simulink model "testsiggen"  (R2018a)
settings: Solver=VariableStepAuto  StartTime=0.0  StopTime=10.0  RelTol=1e-3
model workspace (MAT data in the model file):
  J = 0.14
  p = [-0.0001 0.1 0 0 0.1]
  spe_speed_sdosession = sldodialogs.data.SessionData
  spe_speed_sdosession.Version = '3.0'
  spe_speed_sdosession.Data.ModelName = 'spe_speed'
  spe_speed_sdosession.Data.ToolType = 'ParameterEstimation'
  spe_speed_sdosession.Data.GUIOptions.NoPromptClose = 0
  spe_speed_sdosession.Data.Workspace.LocalWorkspace.EstimationData = sdo.Experiment
  spe_speed_sdosession.Data.Workspace.LocalWorkspace.EstimationData.ModelName = 'spe_speed'
  spe_speed_sdosession.Data.Workspace.LocalWorkspace.EstimationData.InputData = Simulink.SimulationData.Signal
  spe_speed_sdosession.Data.Workspace.LocalWorkspace.EstimationData.InputData.BlockPath = Simulink.SimulationData.BlockPath
  spe_speed_sdosession.Data.Workspace.LocalWorkspace.EstimationData.InputData.BlockPath.path = {'spe_speed/Throttle'}
  spe_speed_sdosession.Data.Workspace.LocalWorkspace.EstimationData.InputData.Values = timeseries
  spe_speed_sdosession.Data.Workspace.LocalWorkspace.EstimationData.InputData.Values.Name = 'spe_speed/Throttle:1'
  spe_speed_sdosession.Data.Workspace.LocalWorkspace.EstimationData.InputData.Values.DataInfo = tsdata.datametadata
  spe_speed_sdosession.Data.Workspace.LocalWorkspace.EstimationData.InputData.Values.DataInfo.Interpolation = tsdata.interpolation
  spe_speed_sdosession.Data.Workspace.LocalWorkspace.EstimationData.InputData.Values.DataInfo.Interpolation.Fhandle : function handle (value not decoded)
  spe_speed_sdosession.Data.Workspace.LocalWorkspace.EstimationData.InputData.Values.DataInfo.Interpolation.Name = 'linear'
  spe_speed_sdosession.Data.Workspace.LocalWorkspace.EstimationData.InputData.Values.TimeInfo = tsdata.timemetadata
  spe_speed_sdosession.Data.Workspace.LocalWorkspace.EstimationData.InputData.Values.TimeInfo.Length = 804
  spe_speed_sdosession.Data.Workspace.LocalWorkspace.EstimationData.InputData.Values.TimeInfo.DuplicateTimes = 0
  spe_speed_sdosession.Data.Workspace.LocalWorkspace.EstimationData.InputData.Values.TimeInfo.Time_ = [0 0.05 0.1 0.15 0.2 0.25 0.3 0.35 0.4 0.45 0.5 0.55 ... (804 elements, 804x1)]
  spe_speed_sdosession.Data.Workspace.LocalWorkspace.EstimationData.InputData.Values.TimeInfo.Initialized = 1
  spe_speed_sdosession.Data.Workspace.LocalWorkspace.EstimationData.InputData.Values.QualityInfo = tsdata.qualmetadata
  spe_speed_sdosession.Data.Workspace.LocalWorkspace.EstimationData.InputData.Values.Data_ = [8.973 8.973 8.973 8.973 8.973 8.973 8.973 8.973 8.973 8.973 8.973 8.973 ... (804 elements, 804x1)]
  spe_speed_sdosession.Data.Workspace.LocalWorkspace.EstimationData.InputData.Name = 'spe_speed/Throttle:1'
  spe_speed_sdosession.Data.Workspace.LocalWorkspace.EstimationData.OutputData = Simulink.SimulationData.Signal
  spe_speed_sdosession.Data.Workspace.LocalWorkspace.EstimationData.OutputData.PortType = 'outport'
  spe_speed_sdosession.Data.Workspace.LocalWorkspace.EstimationData.OutputData.BlockPath = Simulink.SimulationData.BlockPath
  spe_speed_sdosession.Data.Workspace.LocalWorkspace.EstimationData.OutputData.BlockPath.path = {'spe_speed/rad//s to rpm'}
  spe_speed_sdosession.Data.Workspace.LocalWorkspace.EstimationData.OutputData.Values = timeseries
  spe_speed_sdosession.Data.Workspace.LocalWorkspace.EstimationData.OutputData.Values.Name = 'spe_speed/rad//s to rpm:1'
  spe_speed_sdosession.Data.Workspace.LocalWorkspace.EstimationData.OutputData.Values.DataInfo = tsdata.datametadata
  spe_speed_sdosession.Data.Workspace.LocalWorkspace.EstimationData.OutputData.Values.DataInfo.Interpolation = tsdata.interpolation
  spe_speed_sdosession.Data.Workspace.LocalWorkspace.EstimationData.OutputData.Values.DataInfo.Interpolation.Fhandle : function handle (value not decoded)
  spe_speed_sdosession.Data.Workspace.LocalWorkspace.EstimationData.OutputData.Values.DataInfo.Interpolation.Name = 'linear'
  spe_speed_sdosession.Data.Workspace.LocalWorkspace.EstimationData.OutputData.Values.TimeInfo = tsdata.timemetadata
  spe_speed_sdosession.Data.Workspace.LocalWorkspace.EstimationData.OutputData.Values.TimeInfo.Length = 804
  spe_speed_sdosession.Data.Workspace.LocalWorkspace.EstimationData.OutputData.Values.TimeInfo.DuplicateTimes = 0
  spe_speed_sdosession.Data.Workspace.LocalWorkspace.EstimationData.OutputData.Values.TimeInfo.Time_ = [0 0.05 0.1 0.15 0.2 0.25 0.3 0.35 0.4 0.45 0.5 0.55 ... (804 elements, 804x1)]
  spe_speed_sdosession.Data.Workspace.LocalWorkspace.EstimationData.OutputData.Values.TimeInfo.Initialized = 1
  spe_speed_sdosession.Data.Workspace.LocalWorkspace.EstimationData.OutputData.Values.QualityInfo = tsdata.qualmetadata
  spe_speed_sdosession.Data.Workspace.LocalWorkspace.EstimationData.OutputData.Values.Data_ = [2005.2 2032.3 1988.5 2017.4 2002.7 1994.8 1987.6 2001.9 2007.9 2003.5 2007.1 2006.9 ... (804 elements, 804x1)]
  spe_speed_sdosession.Data.Workspace.LocalWorkspace.EstimationData.OutputData.Name = 'spe_speed/rad//s to rpm:1'
  spe_speed_sdosession.Data.Workspace.LocalWorkspace.EstimationData.Name = 'EstimationData'
  spe_speed_sdosession.Data.Workspace.LocalWorkspace.ValidationData = sdo.Experiment
  spe_speed_sdosession.Data.Workspace.LocalWorkspace.ValidationData.ModelName = 'spe_speed'
  spe_speed_sdosession.Data.Workspace.LocalWorkspace.ValidationData.InputData = Simulink.SimulationData.Signal
  spe_speed_sdosession.Data.Workspace.LocalWorkspace.ValidationData.InputData.BlockPath = Simulink.SimulationData.BlockPath
  spe_speed_sdosession.Data.Workspace.LocalWorkspace.ValidationData.InputData.BlockPath.path = {'spe_speed/Throttle'}
  spe_speed_sdosession.Data.Workspace.LocalWorkspace.ValidationData.InputData.Values = timeseries
  spe_speed_sdosession.Data.Workspace.LocalWorkspace.ValidationData.InputData.Values.Name = 'unnamed'
  spe_speed_sdosession.Data.Workspace.LocalWorkspace.ValidationData.InputData.Values.DataInfo = tsdata.datametadata
  spe_speed_sdosession.Data.Workspace.LocalWorkspace.ValidationData.InputData.Values.DataInfo.Interpolation = tsdata.interpolation
  spe_speed_sdosession.Data.Workspace.LocalWorkspace.ValidationData.InputData.Values.DataInfo.Interpolation.Fhandle : function handle (value not decoded)
  spe_speed_sdosession.Data.Workspace.LocalWorkspace.ValidationData.InputData.Values.DataInfo.Interpolation.Name = 'linear'
  spe_speed_sdosession.Data.Workspace.LocalWorkspace.ValidationData.InputData.Values.TimeInfo = tsdata.timemetadata
  spe_speed_sdosession.Data.Workspace.LocalWorkspace.ValidationData.InputData.Values.TimeInfo.Length = 801
  spe_speed_sdosession.Data.Workspace.LocalWorkspace.ValidationData.InputData.Values.TimeInfo.DuplicateTimes = 0
  spe_speed_sdosession.Data.Workspace.LocalWorkspace.ValidationData.InputData.Values.TimeInfo.Time_ = [0 0.05 0.1 0.15 0.2 0.25 0.3 0.35 0.4 0.45 0.5 0.55 ... (801 elements, 801x1)]
  spe_speed_sdosession.Data.Workspace.LocalWorkspace.ValidationData.InputData.Values.TimeInfo.Initialized = 1
  spe_speed_sdosession.Data.Workspace.LocalWorkspace.ValidationData.InputData.Values.QualityInfo = tsdata.qualmetadata
  spe_speed_sdosession.Data.Workspace.LocalWorkspace.ValidationData.InputData.Values.Data_ = [8.973 8.9734 8.974 8.9748 8.9758 8.977 8.9784 8.98 8.9818 8.9838 8.9859 8.9883 ... (801 elements, 801x1)]
  spe_speed_sdosession.Data.Workspace.LocalWorkspace.ValidationData.OutputData = Simulink.SimulationData.Signal
  spe_speed_sdosession.Data.Workspace.LocalWorkspace.ValidationData.OutputData.PortType = 'outport'
  spe_speed_sdosession.Data.Workspace.LocalWorkspace.ValidationData.OutputData.BlockPath = Simulink.SimulationData.BlockPath
  spe_speed_sdosession.Data.Workspace.LocalWorkspace.ValidationData.OutputData.BlockPath.path = {'spe_speed/rad//s to rpm'}
  spe_speed_sdosession.Data.Workspace.LocalWorkspace.ValidationData.OutputData.Values = timeseries
  spe_speed_sdosession.Data.Workspace.LocalWorkspace.ValidationData.OutputData.Values.Name = 'unnamed'
  spe_speed_sdosession.Data.Workspace.LocalWorkspace.ValidationData.OutputData.Values.DataInfo = tsdata.datametadata
  spe_speed_sdosession.Data.Workspace.LocalWorkspace.ValidationData.OutputData.Values.DataInfo.Interpolation = tsdata.interpolation
  spe_speed_sdosession.Data.Workspace.LocalWorkspace.ValidationData.OutputData.Values.DataInfo.Interpolation.Fhandle : function handle (value not decoded)
  spe_speed_sdosession.Data.Workspace.LocalWorkspace.ValidationData.OutputData.Values.DataInfo.Interpolation.Name = 'linear'
  spe_speed_sdosession.Data.Workspace.LocalWorkspace.ValidationData.OutputData.Values.TimeInfo = tsdata.timemetadata
  spe_speed_sdosession.Data.Workspace.LocalWorkspace.ValidationData.OutputData.Values.TimeInfo.Length = 801
  spe_speed_sdosession.Data.Workspace.LocalWorkspace.ValidationData.OutputData.Values.TimeInfo.DuplicateTimes = 0
  spe_speed_sdosession.Data.Workspace.LocalWorkspace.ValidationData.OutputData.Values.TimeInfo.Time_ = [0 0.05 0.1 0.15 0.2 0.25 0.3 0.35 0.4 0.45 0.5 0.55 ... (801 elements, 801x1)]
  spe_speed_sdosession.Data.Workspace.LocalWorkspace.ValidationData.OutputData.Values.TimeInfo.Initialized = 1
  spe_speed_sdosession.Data.Workspace.LocalWorkspace.ValidationData.OutputData.Values.QualityInfo = tsdata.qualmetadata
  spe_speed_sdosession.Data.Workspace.LocalWorkspace.ValidationData.OutputData.Values.Data_ = [2005.2 2032.3 1988.5 2017.4 2002.7 1994.9 1987.8 2002.1 2008.2 2004 2007.7 2007.7 ... (801 elements, 801x1)]
  spe_speed_sdosession.Data.Workspace.LocalWorkspace.ValidationData.Name = 'ValidationData'
  spe_speed_sdosession.Data.Workspace.HiddenWorkspace.EstimatedParams = param.Continuous
  spe_speed_sdosession.Data.Workspace.HiddenWorkspace.EstimatedParams.Scale_ = [-0.0001 0.1 0 0 0.1]
  spe_speed_sdosession.Data.Workspace.HiddenWorkspace.EstimatedParams.Size_ = [1 5]
  spe_speed_sdosession.Data.Workspace.HiddenWorkspace.EstimatedParams.Value_ = [-0.0001 0.1 0 0 0.1]
  spe_speed_sdosession.Data.Workspace.HiddenWorkspace.EstimatedParams.pID = paramid.Variable
  spe_speed_sdosession.Data.Workspace.HiddenWorkspace.EstimatedParams.pID.Name = 'p'
  spe_speed_sdosession.Data.Workspace.HiddenWorkspace.UVars = []
  spe_speed_sdosession.Data.ToolData.PlotManager.Plots.Class = 'sldoplots.ExperimentPlot'
  spe_speed_sdosession.Data.ToolData.PlotManager.Plots.Sources = {'EstimationData'}
  spe_speed_sdosession.Data.ToolData.DialogManager = []
  spe_speed_sdosession.Data.ToolData.ParameterEstimation.DesignVariables = 'EstimatedParams'
  spe_speed_sdosession.Data.ToolData.ParameterEstimation.UncertainVariables = 'UVars'
  spe_speed_sdosession.Data.ToolData.ParameterEstimation.Options = sdo.OptimizeOptions
  spe_speed_sdosession.Data.ToolData.ParameterEstimation.Options.Method = 'lsqnonlin'
  spe_speed_sdosession.Data.ToolData.ParameterEstimation.Options.MethodOptions = optim.options.Lsqnonlin
  spe_speed_sdosession.Data.ToolData.ParameterEstimation.Options.MethodOptions.LsqnonlinVersion = 4
  spe_speed_sdosession.Data.ToolData.ParameterEstimation.Options.MethodOptions.OptionsStore.AlgorithmNames = {'trust-region-reflective', 'levenberg-marquardt'}
  spe_speed_sdosession.Data.ToolData.ParameterEstimation.Options.MethodOptions.OptionsStore.DefaultAlgorithm = 'trust-region-reflective'
  spe_speed_sdosession.Data.ToolData.ParameterEstimation.Options.MethodOptions.OptionsStore.AlgorithmDefaults{1}.DerivativeCheck = 'off'
  spe_speed_sdosession.Data.ToolData.ParameterEstimation.Options.MethodOptions.OptionsStore.AlgorithmDefaults{1}.Diagnostics = 'off'
  spe_speed_sdosession.Data.ToolData.ParameterEstimation.Options.MethodOptions.OptionsStore.AlgorithmDefaults{1}.DiffMaxChange = Inf
  spe_speed_sdosession.Data.ToolData.ParameterEstimation.Options.MethodOptions.OptionsStore.AlgorithmDefaults{1}.DiffMinChange = 0
  spe_speed_sdosession.Data.ToolData.ParameterEstimation.Options.MethodOptions.OptionsStore.AlgorithmDefaults{1}.Display = 'final'
  spe_speed_sdosession.Data.ToolData.ParameterEstimation.Options.MethodOptions.OptionsStore.AlgorithmDefaults{1}.FinDiffRelStep = 'sqrt(eps)'
  spe_speed_sdosession.Data.ToolData.ParameterEstimation.Options.MethodOptions.OptionsStore.AlgorithmDefaults{1}.FinDiffType = 'forward'
  spe_speed_sdosession.Data.ToolData.ParameterEstimation.Options.MethodOptions.OptionsStore.AlgorithmDefaults{1}.FunValCheck = 'off'
  spe_speed_sdosession.Data.ToolData.ParameterEstimation.Options.MethodOptions.OptionsStore.AlgorithmDefaults{1}.Jacobian = 'off'
  spe_speed_sdosession.Data.ToolData.ParameterEstimation.Options.MethodOptions.OptionsStore.AlgorithmDefaults{1}.MaxFunEvals = '100*numberOfVariables'
  spe_speed_sdosession.Data.ToolData.ParameterEstimation.Options.MethodOptions.OptionsStore.AlgorithmDefaults{1}.MaxIter = 400
  spe_speed_sdosession.Data.ToolData.ParameterEstimation.Options.MethodOptions.OptionsStore.AlgorithmDefaults{1}.OutputFcn = []
  spe_speed_sdosession.Data.ToolData.ParameterEstimation.Options.MethodOptions.OptionsStore.AlgorithmDefaults{1}.PlotFcns = []
  spe_speed_sdosession.Data.ToolData.ParameterEstimation.Options.MethodOptions.OptionsStore.AlgorithmDefaults{1}.TolFunValue = 1e-06
  spe_speed_sdosession.Data.ToolData.ParameterEstimation.Options.MethodOptions.OptionsStore.AlgorithmDefaults{1}.TolFun = 1e-06
  spe_speed_sdosession.Data.ToolData.ParameterEstimation.Options.MethodOptions.OptionsStore.AlgorithmDefaults{1}.TolX = 1e-06
  spe_speed_sdosession.Data.ToolData.ParameterEstimation.Options.MethodOptions.OptionsStore.AlgorithmDefaults{1}.TypicalX = 'ones(numberOfVariables,1)'
  spe_speed_sdosession.Data.ToolData.ParameterEstimation.Options.MethodOptions.OptionsStore.AlgorithmDefaults{1}.JacobMult = []
  spe_speed_sdosession.Data.ToolData.ParameterEstimation.Options.MethodOptions.OptionsStore.AlgorithmDefaults{1}.JacobPattern = 'sparse(ones(Jrows,Jcols))'
  spe_speed_sdosession.Data.ToolData.ParameterEstimation.Options.MethodOptions.OptionsStore.AlgorithmDefaults{1}.MaxPCGIter = 'max(1,floor(numberOfVariables/2))'
  spe_speed_sdosession.Data.ToolData.ParameterEstimation.Options.MethodOptions.OptionsStore.AlgorithmDefaults{1}.PrecondBandWidth = Inf
  spe_speed_sdosession.Data.ToolData.ParameterEstimation.Options.MethodOptions.OptionsStore.AlgorithmDefaults{1}.TolPCG = 0.1
  spe_speed_sdosession.Data.ToolData.ParameterEstimation.Options.MethodOptions.OptionsStore.AlgorithmDefaults{1}.UseParallel = 0
  spe_speed_sdosession.Data.ToolData.ParameterEstimation.Options.MethodOptions.OptionsStore.AlgorithmDefaults{2}.DerivativeCheck = 'off'
  spe_speed_sdosession.Data.ToolData.ParameterEstimation.Options.MethodOptions.OptionsStore.AlgorithmDefaults{2}.Diagnostics = 'off'
  spe_speed_sdosession.Data.ToolData.ParameterEstimation.Options.MethodOptions.OptionsStore.AlgorithmDefaults{2}.DiffMaxChange = Inf
  spe_speed_sdosession.Data.ToolData.ParameterEstimation.Options.MethodOptions.OptionsStore.AlgorithmDefaults{2}.DiffMinChange = 0
  spe_speed_sdosession.Data.ToolData.ParameterEstimation.Options.MethodOptions.OptionsStore.AlgorithmDefaults{2}.Display = 'final'
  spe_speed_sdosession.Data.ToolData.ParameterEstimation.Options.MethodOptions.OptionsStore.AlgorithmDefaults{2}.FinDiffRelStep = 'sqrt(eps)'
  spe_speed_sdosession.Data.ToolData.ParameterEstimation.Options.MethodOptions.OptionsStore.AlgorithmDefaults{2}.FinDiffType = 'forward'
  spe_speed_sdosession.Data.ToolData.ParameterEstimation.Options.MethodOptions.OptionsStore.AlgorithmDefaults{2}.FunValCheck = 'off'
  spe_speed_sdosession.Data.ToolData.ParameterEstimation.Options.MethodOptions.OptionsStore.AlgorithmDefaults{2}.Jacobian = 'off'
  spe_speed_sdosession.Data.ToolData.ParameterEstimation.Options.MethodOptions.OptionsStore.AlgorithmDefaults{2}.InitDamping = 0.01
  spe_speed_sdosession.Data.ToolData.ParameterEstimation.Options.MethodOptions.OptionsStore.AlgorithmDefaults{2}.MaxFunEvals = '200*numberOfVariables'
  spe_speed_sdosession.Data.ToolData.ParameterEstimation.Options.MethodOptions.OptionsStore.AlgorithmDefaults{2}.MaxIter = 400
  spe_speed_sdosession.Data.ToolData.ParameterEstimation.Options.MethodOptions.OptionsStore.AlgorithmDefaults{2}.OutputFcn = []
  spe_speed_sdosession.Data.ToolData.ParameterEstimation.Options.MethodOptions.OptionsStore.AlgorithmDefaults{2}.PlotFcns = []
  spe_speed_sdosession.Data.ToolData.ParameterEstimation.Options.MethodOptions.OptionsStore.AlgorithmDefaults{2}.TolFunValue = 1e-06
  spe_speed_sdosession.Data.ToolData.ParameterEstimation.Options.MethodOptions.OptionsStore.AlgorithmDefaults{2}.TolX = 1e-06
  spe_speed_sdosession.Data.ToolData.ParameterEstimation.Options.MethodOptions.OptionsStore.AlgorithmDefaults{2}.TypicalX = 'ones(numberOfVariables,1)'
  spe_speed_sdosession.Data.ToolData.ParameterEstimation.Options.MethodOptions.OptionsStore.AlgorithmDefaults{2}.ScaleProblem = 'none'
  spe_speed_sdosession.Data.ToolData.ParameterEstimation.Options.MethodOptions.OptionsStore.AlgorithmDefaults{2}.UseParallel = 0
  spe_speed_sdosession.Data.ToolData.ParameterEstimation.Options.MethodOptions.OptionsStore.AlgorithmIndex = [1 0]
  spe_speed_sdosession.Data.ToolData.ParameterEstimation.Options.MethodOptions.OptionsStore.SetByUser.DerivativeCheck = 0
  spe_speed_sdosession.Data.ToolData.ParameterEstimation.Options.MethodOptions.OptionsStore.SetByUser.Diagnostics = 0
  spe_speed_sdosession.Data.ToolData.ParameterEstimation.Options.MethodOptions.OptionsStore.SetByUser.DiffMaxChange = 0
  spe_speed_sdosession.Data.ToolData.ParameterEstimation.Options.MethodOptions.OptionsStore.SetByUser.DiffMinChange = 0
  spe_speed_sdosession.Data.ToolData.ParameterEstimation.Options.MethodOptions.OptionsStore.SetByUser.Display = 1
  spe_speed_sdosession.Data.ToolData.ParameterEstimation.Options.MethodOptions.OptionsStore.SetByUser.FinDiffRelStep = 0
  spe_speed_sdosession.Data.ToolData.ParameterEstimation.Options.MethodOptions.OptionsStore.SetByUser.FinDiffType = 0
  spe_speed_sdosession.Data.ToolData.ParameterEstimation.Options.MethodOptions.OptionsStore.SetByUser.FunValCheck = 0
  spe_speed_sdosession.Data.ToolData.ParameterEstimation.Options.MethodOptions.OptionsStore.SetByUser.InitDamping = 0
  spe_speed_sdosession.Data.ToolData.ParameterEstimation.Options.MethodOptions.OptionsStore.SetByUser.JacobMult = 0
  spe_speed_sdosession.Data.ToolData.ParameterEstimation.Options.MethodOptions.OptionsStore.SetByUser.JacobPattern = 0
  spe_speed_sdosession.Data.ToolData.ParameterEstimation.Options.MethodOptions.OptionsStore.SetByUser.Jacobian = 1
  spe_speed_sdosession.Data.ToolData.ParameterEstimation.Options.MethodOptions.OptionsStore.SetByUser.MaxFunEvals = 1
  spe_speed_sdosession.Data.ToolData.ParameterEstimation.Options.MethodOptions.OptionsStore.SetByUser.MaxIter = 1
  spe_speed_sdosession.Data.ToolData.ParameterEstimation.Options.MethodOptions.OptionsStore.SetByUser.MaxPCGIter = 0
  spe_speed_sdosession.Data.ToolData.ParameterEstimation.Options.MethodOptions.OptionsStore.SetByUser.OutputFcn = 0
  spe_speed_sdosession.Data.ToolData.ParameterEstimation.Options.MethodOptions.OptionsStore.SetByUser.PlotFcns = 0
  spe_speed_sdosession.Data.ToolData.ParameterEstimation.Options.MethodOptions.OptionsStore.SetByUser.PrecondBandWidth = 0
  spe_speed_sdosession.Data.ToolData.ParameterEstimation.Options.MethodOptions.OptionsStore.SetByUser.ScaleProblem = 0
  spe_speed_sdosession.Data.ToolData.ParameterEstimation.Options.MethodOptions.OptionsStore.SetByUser.TolFun = 1
  spe_speed_sdosession.Data.ToolData.ParameterEstimation.Options.MethodOptions.OptionsStore.SetByUser.TolFunValue = 1
  spe_speed_sdosession.Data.ToolData.ParameterEstimation.Options.MethodOptions.OptionsStore.SetByUser.TolPCG = 0
  spe_speed_sdosession.Data.ToolData.ParameterEstimation.Options.MethodOptions.OptionsStore.SetByUser.TolX = 1
  spe_speed_sdosession.Data.ToolData.ParameterEstimation.Options.MethodOptions.OptionsStore.SetByUser.TypicalX = 0
  spe_speed_sdosession.Data.ToolData.ParameterEstimation.Options.MethodOptions.OptionsStore.SetByUser.UseParallel = 0
  spe_speed_sdosession.Data.ToolData.ParameterEstimation.Options.MethodOptions.OptionsStore.SetByUser.Algorithm = 0
  spe_speed_sdosession.Data.ToolData.ParameterEstimation.Options.MethodOptions.OptionsStore.NonConstantDefaultFields = {'MaxFunEvals'}
  spe_speed_sdosession.Data.ToolData.ParameterEstimation.Options.MethodOptions.OptionsStore.IsConstantDefault.DerivativeCheck = 1
  spe_speed_sdosession.Data.ToolData.ParameterEstimation.Options.MethodOptions.OptionsStore.IsConstantDefault.Diagnostics = 1
  spe_speed_sdosession.Data.ToolData.ParameterEstimation.Options.MethodOptions.OptionsStore.IsConstantDefault.DiffMaxChange = 1
  spe_speed_sdosession.Data.ToolData.ParameterEstimation.Options.MethodOptions.OptionsStore.IsConstantDefault.DiffMinChange = 1
  spe_speed_sdosession.Data.ToolData.ParameterEstimation.Options.MethodOptions.OptionsStore.IsConstantDefault.Display = 1
  spe_speed_sdosession.Data.ToolData.ParameterEstimation.Options.MethodOptions.OptionsStore.IsConstantDefault.FinDiffRelStep = 1
  spe_speed_sdosession.Data.ToolData.ParameterEstimation.Options.MethodOptions.OptionsStore.IsConstantDefault.FinDiffType = 1
  spe_speed_sdosession.Data.ToolData.ParameterEstimation.Options.MethodOptions.OptionsStore.IsConstantDefault.FunValCheck = 1
  spe_speed_sdosession.Data.ToolData.ParameterEstimation.Options.MethodOptions.OptionsStore.IsConstantDefault.InitDamping = 1
  spe_speed_sdosession.Data.ToolData.ParameterEstimation.Options.MethodOptions.OptionsStore.IsConstantDefault.JacobMult = 1
  spe_speed_sdosession.Data.ToolData.ParameterEstimation.Options.MethodOptions.OptionsStore.IsConstantDefault.JacobPattern = 1
  spe_speed_sdosession.Data.ToolData.ParameterEstimation.Options.MethodOptions.OptionsStore.IsConstantDefault.Jacobian = 1
  spe_speed_sdosession.Data.ToolData.ParameterEstimation.Options.MethodOptions.OptionsStore.IsConstantDefault.MaxFunEvals = 0
  spe_speed_sdosession.Data.ToolData.ParameterEstimation.Options.MethodOptions.OptionsStore.IsConstantDefault.MaxIter = 1
  spe_speed_sdosession.Data.ToolData.ParameterEstimation.Options.MethodOptions.OptionsStore.IsConstantDefault.MaxPCGIter = 1
  spe_speed_sdosession.Data.ToolData.ParameterEstimation.Options.MethodOptions.OptionsStore.IsConstantDefault.OutputFcn = 1
  spe_speed_sdosession.Data.ToolData.ParameterEstimation.Options.MethodOptions.OptionsStore.IsConstantDefault.PlotFcns = 1
  spe_speed_sdosession.Data.ToolData.ParameterEstimation.Options.MethodOptions.OptionsStore.IsConstantDefault.PrecondBandWidth = 1
  spe_speed_sdosession.Data.ToolData.ParameterEstimation.Options.MethodOptions.OptionsStore.IsConstantDefault.ScaleProblem = 1
  spe_speed_sdosession.Data.ToolData.ParameterEstimation.Options.MethodOptions.OptionsStore.IsConstantDefault.TolFun = 1
  spe_speed_sdosession.Data.ToolData.ParameterEstimation.Options.MethodOptions.OptionsStore.IsConstantDefault.TolFunValue = 1
  spe_speed_sdosession.Data.ToolData.ParameterEstimation.Options.MethodOptions.OptionsStore.IsConstantDefault.TolPCG = 1
  spe_speed_sdosession.Data.ToolData.ParameterEstimation.Options.MethodOptions.OptionsStore.IsConstantDefault.TolX = 1
  spe_speed_sdosession.Data.ToolData.ParameterEstimation.Options.MethodOptions.OptionsStore.IsConstantDefault.TypicalX = 1
  spe_speed_sdosession.Data.ToolData.ParameterEstimation.Options.MethodOptions.OptionsStore.IsConstantDefault.UseParallel = 1
  spe_speed_sdosession.Data.ToolData.ParameterEstimation.Options.MethodOptions.OptionsStore.IsConstantDefault.Algorithm = 1
  spe_speed_sdosession.Data.ToolData.ParameterEstimation.Options.MethodOptions.OptionsStore.NonConstantDefaults.MaxFunEvals = {'100*numberOfVariables', '200*numberOfVariables'}
  spe_speed_sdosession.Data.ToolData.ParameterEstimation.Options.MethodOptions.OptionsStore.Options.DerivativeCheck = 'off'
  spe_speed_sdosession.Data.ToolData.ParameterEstimation.Options.MethodOptions.OptionsStore.Options.Diagnostics = 'off'
  spe_speed_sdosession.Data.ToolData.ParameterEstimation.Options.MethodOptions.OptionsStore.Options.DiffMaxChange = Inf
  spe_speed_sdosession.Data.ToolData.ParameterEstimation.Options.MethodOptions.OptionsStore.Options.DiffMinChange = 0
  spe_speed_sdosession.Data.ToolData.ParameterEstimation.Options.MethodOptions.OptionsStore.Options.Display = 'iter'
  spe_speed_sdosession.Data.ToolData.ParameterEstimation.Options.MethodOptions.OptionsStore.Options.FinDiffRelStep = 'sqrt(eps)'
  spe_speed_sdosession.Data.ToolData.ParameterEstimation.Options.MethodOptions.OptionsStore.Options.FinDiffType = 'forward'
  spe_speed_sdosession.Data.ToolData.ParameterEstimation.Options.MethodOptions.OptionsStore.Options.FunValCheck = 'off'
  spe_speed_sdosession.Data.ToolData.ParameterEstimation.Options.MethodOptions.OptionsStore.Options.Jacobian = 'on'
  spe_speed_sdosession.Data.ToolData.ParameterEstimation.Options.MethodOptions.OptionsStore.Options.MaxFunEvals = Inf
  spe_speed_sdosession.Data.ToolData.ParameterEstimation.Options.MethodOptions.OptionsStore.Options.MaxIter = 100
  spe_speed_sdosession.Data.ToolData.ParameterEstimation.Options.MethodOptions.OptionsStore.Options.OutputFcn = []
  spe_speed_sdosession.Data.ToolData.ParameterEstimation.Options.MethodOptions.OptionsStore.Options.PlotFcns = []
  spe_speed_sdosession.Data.ToolData.ParameterEstimation.Options.MethodOptions.OptionsStore.Options.TolFunValue = 1e-06
  spe_speed_sdosession.Data.ToolData.ParameterEstimation.Options.MethodOptions.OptionsStore.Options.TolFun = 1e-06
  spe_speed_sdosession.Data.ToolData.ParameterEstimation.Options.MethodOptions.OptionsStore.Options.TolX = 1e-06
  spe_speed_sdosession.Data.ToolData.ParameterEstimation.Options.MethodOptions.OptionsStore.Options.TypicalX = 'ones(numberOfVariables,1)'
  spe_speed_sdosession.Data.ToolData.ParameterEstimation.Options.MethodOptions.OptionsStore.Options.JacobMult = []
  spe_speed_sdosession.Data.ToolData.ParameterEstimation.Options.MethodOptions.OptionsStore.Options.JacobPattern = 'sparse(ones(Jrows,Jcols))'
  spe_speed_sdosession.Data.ToolData.ParameterEstimation.Options.MethodOptions.OptionsStore.Options.MaxPCGIter = 'max(1,floor(numberOfVariables/2))'
  spe_speed_sdosession.Data.ToolData.ParameterEstimation.Options.MethodOptions.OptionsStore.Options.PrecondBandWidth = Inf
  spe_speed_sdosession.Data.ToolData.ParameterEstimation.Options.MethodOptions.OptionsStore.Options.TolPCG = 0.1
  spe_speed_sdosession.Data.ToolData.ParameterEstimation.Options.MethodOptions.OptionsStore.Options.UseParallel = 0
  spe_speed_sdosession.Data.ToolData.ParameterEstimation.Options.MethodOptions.OptionsStore.Options.InitDamping = 0.01
  spe_speed_sdosession.Data.ToolData.ParameterEstimation.Options.MethodOptions.OptionsStore.Options.ScaleProblem = 'none'
  spe_speed_sdosession.Data.ToolData.ParameterEstimation.Options.MethodOptions.OptionsStore.Options.Algorithm = 'trust-region-reflective'
  spe_speed_sdosession.Data.ToolData.ParameterEstimation.Options.MethodOptions.OptionsStore.NumDisplayOptions = [17 14]
  spe_speed_sdosession.Data.ToolData.ParameterEstimation.Options.MethodOptions.OptionsStore.DisplayOptions = {{'CheckGradients', 'Display', 'FiniteDifferenceStepSize', 'FiniteDifferenceType', 'SpecifyObjectiveGradient', 'MaxFunctionEvaluations', 'MaxIterations', 'OutputFcn', 'PlotFcn', 'FunctionTolerance', 'OptimalityTolerance', 'StepTolerance', 'TypicalX', 'JacobianMultiplyFcn', 'SubproblemAlgorithm', 'UseParallel', 'Algorithm'}, {'CheckGradients', 'Display', 'FiniteDifferenceStepSize', 'FiniteDifferenceType', 'SpecifyObjectiveGradient', 'MaxFunctionEvaluations', 'MaxIterations', 'OutputFcn', 'PlotFcn', 'FunctionTolerance', 'StepTolerance', 'TypicalX', 'UseParallel', 'Algorithm'}}
  spe_speed_sdosession.Data.ToolData.ParameterEstimation.Options.MethodOptions.Version = 2
  spe_speed_sdosession.Data.ToolData.ParameterEstimation.Options.OptimizedModel = 'spe_speed'
  spe_speed_sdosession.Data.ToolData.ParameterEstimation.GUIOptions.ShowProgress = 1
  spe_speed_sdosession.Data.ToolData.ParameterEstimation.GUIOptions.UpdatePlots = 1
  spe_speed_sdosession.Data.ToolData.ParameterEstimation.GUIOptions.UpdateModel = 1
  spe_speed_sdosession.Data.ToolData.ParameterEstimation.GUIOptions.UpdateDesign = 'overwrite'
  spe_speed_sdosession.Data.ToolData.ParameterEstimation.GUIOptions.SaveReport = 0
  spe_speed_sdosession.Data.ToolData.ParameterEstimation.GUIOptions.SaveRequirementValue = 1
  spe_speed_sdosession.Data.ToolData.ParameterEstimation.DataToPlot = ''
  spe_speed_sdosession.Data.ToolData.ParameterEstimation.LocalRequirements = struct([])
  spe_speed_sdosession.Data.ToolData.ParameterEstimation.BlockRequirements = struct([])
  spe_speed_sdosession.Data.ToolData.ParameterEstimation.LocalExperiments(1).SelectedForEstimation = 1
  spe_speed_sdosession.Data.ToolData.ParameterEstimation.LocalExperiments(1).SelectedForValidation = 0
  spe_speed_sdosession.Data.ToolData.ParameterEstimation.LocalExperiments(1).Experiment = 'EstimationData'
  spe_speed_sdosession.Data.ToolData.ParameterEstimation.LocalExperiments(2).SelectedForEstimation = 0
  spe_speed_sdosession.Data.ToolData.ParameterEstimation.LocalExperiments(2).SelectedForValidation = 0
  spe_speed_sdosession.Data.ToolData.ParameterEstimation.LocalExperiments(2).Experiment = 'ValidationData'
  spe_speed_sdosession.Data.ToolData.ParameterEstimation.LocalResults.SelectedForValidation = 1
  spe_speed_sdosession.Data.ToolData.ParameterEstimation.LocalResults.Result = 'Use current parameter values'
  spe_speed_sdosession.Data.ToolData.ParameterEstimation.Cost.Type = 'SSE'
  spe_speed_sdosession.Data.ToolData.ParameterEstimation.Cost.Robust = 'off'
  speed1 = [2005.2 2032.3 1988.5 2017.4 2002.7 1994.8 1987.6 2001.9 2007.9 2003.5 2007.1 2006.9 ... (804 elements, 804x1)]
  speed2 = [2005.2 2032.3 1988.5 2017.4 2002.7 1994.9 1987.8 2002.1 2008.2 2004 2007.7 2007.7 ... (801 elements, 801x1)]
  throttle1 = [8.973 8.973 8.973 8.973 8.973 8.973 8.973 8.973 8.973 8.973 8.973 8.973 ... (804 elements, 804x1)]
  throttle2 = [8.973 8.9734 8.974 8.9748 8.9758 8.977 8.9784 8.98 8.9818 8.9838 8.9859 8.9883 ... (801 elements, 801x1)]
  time1 = [0 0.05 0.1 0.15 0.2 0.25 0.3 0.35 0.4 0.45 0.5 0.55 ... (804 elements, 804x1)]
  time2 = [0 0.05 0.1 0.15 0.2 0.25 0.3 0.35 0.4 0.45 0.5 0.55 ... (801 elements, 801x1)]
libraries: dspxfrm3 x1, simulink x1
settings Model: Creator=Thinkpad  LastModifiedBy=Thinkpad

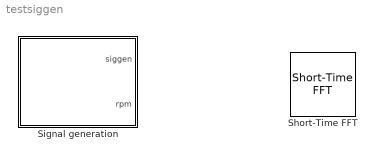
== system testsiggen ==
  Short-Time FFT : dspxfrm3/Short-Time FFT  W=512  OvLap=384  M=1024
      settings: SourceProductName=DSP System Toolbox  SourceProductBaseCode=DS
  Signal generation : Subsystem

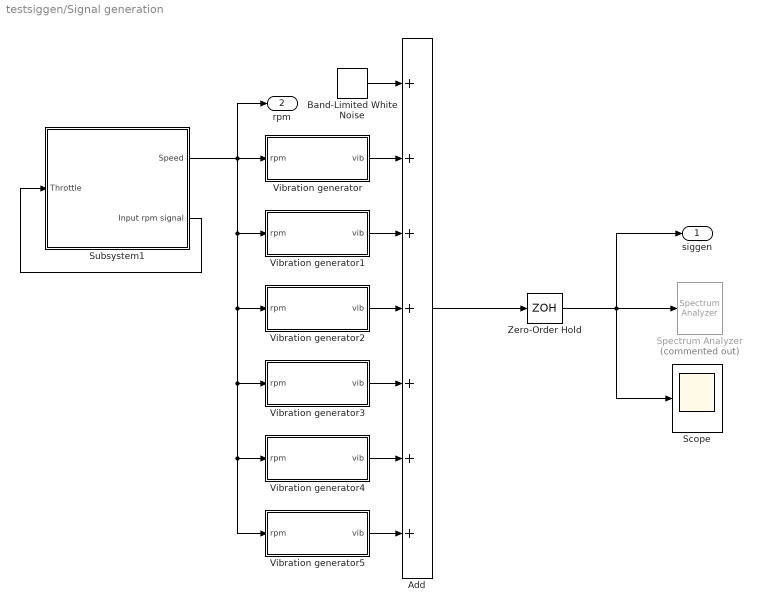
== system testsiggen/Signal generation ==
  Add : Sum  Inputs=+++++++
  Band-Limited White Noise : simulink/Sources/Band-Limited White Noise  Cov=[1e-5]  Ts=1e-5  seed=[23341]
  Scope : Scope
  Spectrum Analyzer : SpectrumAnalyzer  Commented=on
  Subsystem1 : Subsystem
  Vibration generator : Subsystem  mask{T=10, order=1}
  Vibration generator1 : Subsystem  mask{T=10, order=3}
  Vibration generator2 : Subsystem  mask{T=10, order=7.2}
  Vibration generator3 : Subsystem  mask{T=10, order=2}
  Vibration generator4 : Subsystem  mask{T=10, order=10}
  Vibration generator5 : Subsystem  mask{T=10, order=4.3}
  Zero-Order Hold : ZeroOrderHold  SampleTime=1e-5
  siggen : Outport
  rpm : Outport  Port=2
  wires:
  Zero-Order Hold/1 -> siggen/1, Scope/1, Spectrum Analyzer/1
  Band-Limited White Noise/1 -> Add/1
  Vibration generator4/1(vib) -> Add/6
  Vibration generator3/1(vib) -> Add/5
  Subsystem1/1(Speed) -> rpm/1, Vibration generator5/1(rpm), Vibration generator4/1(rpm), Vibration generator3/1(rpm), Vibration generator2/1(rpm), Vibration generator1/1(rpm), Vibration generator/1(rpm)
  Vibration generator/1(vib) -> Add/2
  Vibration generator1/1(vib) -> Add/3
  Vibration generator2/1(vib) -> Add/4
  Vibration generator5/1(vib) -> Add/7
  Add/1 -> Zero-Order Hold/1
  Subsystem1/2(Input rpm signal) -> Subsystem1/1(Throttle)

== system testsiggen/Signal generation/Subsystem1 ==
  Throttle : Inport
  Engine Speed (rpm) : Scope
  Engine speed model : Subsystem
  Manual Switch : ManualSwitch
  Throttle (degrees) : Step  Time=2  Before=8.973  After=11  SampleTime=0
  Speed : Outport
  Input rpm signal : Outport  Port=2
  wires:
  Manual Switch/1 -> Engine speed model/1(Throttle)
  Throttle/1 -> Manual Switch/2
  Throttle (degrees)/1 -> Manual Switch/1
  Engine speed model/1(Speed) -> Engine Speed (rpm)/1, Input rpm signal/1, Speed/1

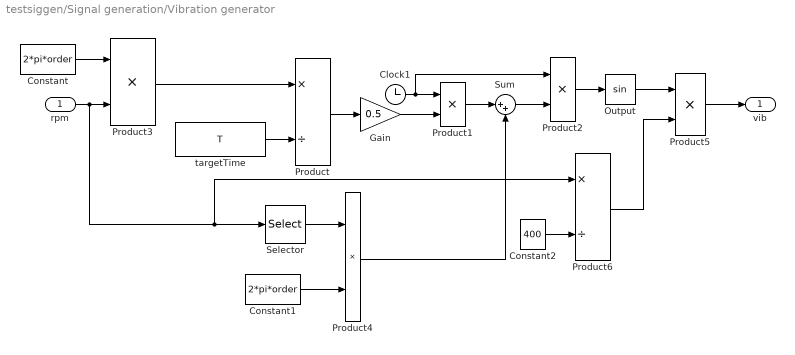
== system testsiggen/Signal generation/Vibration generator ==
  rpm : Inport
  Clock1 : Clock
      settings: DisableCoverage=on
  Constant : Constant  Value=2*pi*order
  Constant1 : Constant  Value=2*pi*order
  Constant2 : Constant  Value=400
  Gain : Gain  DisableCoverage=on  Gain=0.5  OutDataTypeStr=Inherit: Same as input  ParamDataTypeStr=Inherit: Same as input
  Output : Trigonometry
  Product : Product  DisableCoverage=on  Inputs=*/  SaturateOnIntegerOverflow=on  InputSameDT=on  OutDataTypeStr=Inherit: Same as first input
  Product1 : Product  DisableCoverage=on  SaturateOnIntegerOverflow=on  InputSameDT=on  OutDataTypeStr=Inherit: Same as first input
  Product2 : Product  DisableCoverage=on  SaturateOnIntegerOverflow=on  InputSameDT=on  OutDataTypeStr=Inherit: Same as first input
  Product3 : Product
  Product4 : Product
  Product5 : Product
  Product6 : Product  DisableCoverage=on  Inputs=*/  SaturateOnIntegerOverflow=on  InputSameDT=on  OutDataTypeStr=Inherit: Same as first input
  Selector : Selector  InputPortWidth=1  IndexOptions=Index vector (dialog)  Indices=[1]  OutputSizes=1
  Sum : Sum  DisableCoverage=on  Inputs=|++  SaturateOnIntegerOverflow=on  InputSameDT=on  OutDataTypeStr=Inherit: Same as first input
  targetTime : Constant  DisableCoverage=on  Value=T
  vib : Outport
  wires:
  Sum/1 -> Product2/2
  targetTime/1 -> Product/2
  Clock1/1 -> Product2/1, Product1/1
  Gain/1 -> Product1/2
  Product2/1 -> Output/1
  Product/1 -> Gain/1
  Product3/1 -> Product/1
  Product1/1 -> Sum/1
  rpm/1 -> Product6/1, Selector/1, Product3/2
  Constant/1 -> Product3/1
  Selector/1 -> Product4/1
  Constant1/1 -> Product4/2
  Product4/1 -> Sum/2
  Output/1 -> Product5/1
  Product5/1 -> vib/1
  Constant2/1 -> Product6/2
  Product6/1 -> Product5/2

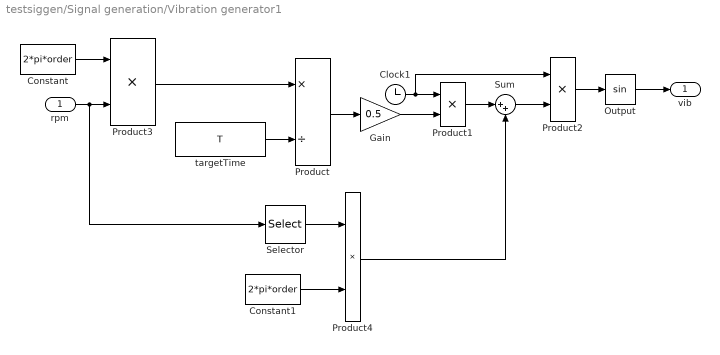
== system testsiggen/Signal generation/Vibration generator1 ==
  rpm : Inport
  Clock1 : Clock
      settings: DisableCoverage=on
  Constant : Constant  Value=2*pi*order
  Constant1 : Constant  Value=2*pi*order
  Gain : Gain  DisableCoverage=on  Gain=0.5  OutDataTypeStr=Inherit: Same as input  ParamDataTypeStr=Inherit: Same as input
  Output : Trigonometry
  Product : Product  DisableCoverage=on  Inputs=*/  SaturateOnIntegerOverflow=on  InputSameDT=on  OutDataTypeStr=Inherit: Same as first input
  Product1 : Product  DisableCoverage=on  SaturateOnIntegerOverflow=on  InputSameDT=on  OutDataTypeStr=Inherit: Same as first input
  Product2 : Product  DisableCoverage=on  SaturateOnIntegerOverflow=on  InputSameDT=on  OutDataTypeStr=Inherit: Same as first input
  Product3 : Product
  Product4 : Product
  Selector : Selector  InputPortWidth=1  IndexOptions=Index vector (dialog)  Indices=[1]  OutputSizes=1
  Sum : Sum  DisableCoverage=on  Inputs=|++  SaturateOnIntegerOverflow=on  InputSameDT=on  OutDataTypeStr=Inherit: Same as first input
  targetTime : Constant  DisableCoverage=on  Value=T
  vib : Outport
  wires:
  Sum/1 -> Product2/2
  targetTime/1 -> Product/2
  Output/1 -> vib/1
  Clock1/1 -> Product2/1, Product1/1
  Gain/1 -> Product1/2
  Product2/1 -> Output/1
  Product/1 -> Gain/1
  Product3/1 -> Product/1
  Product1/1 -> Sum/1
  rpm/1 -> Selector/1, Product3/2
  Constant/1 -> Product3/1
  Selector/1 -> Product4/1
  Constant1/1 -> Product4/2
  Product4/1 -> Sum/2

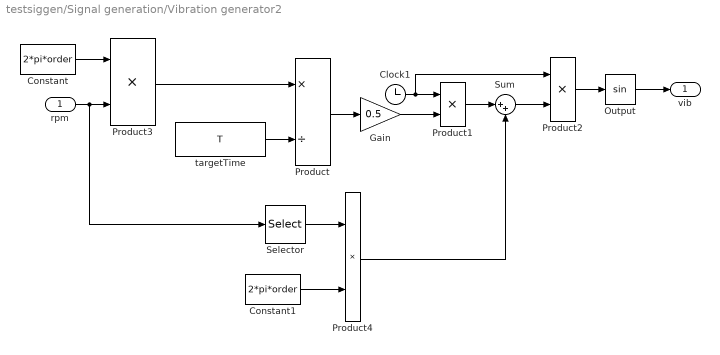
== system testsiggen/Signal generation/Vibration generator2 ==
  rpm : Inport
  Clock1 : Clock
      settings: DisableCoverage=on
  Constant : Constant  Value=2*pi*order
  Constant1 : Constant  Value=2*pi*order
  Gain : Gain  DisableCoverage=on  Gain=0.5  OutDataTypeStr=Inherit: Same as input  ParamDataTypeStr=Inherit: Same as input
  Output : Trigonometry
  Product : Product  DisableCoverage=on  Inputs=*/  SaturateOnIntegerOverflow=on  InputSameDT=on  OutDataTypeStr=Inherit: Same as first input
  Product1 : Product  DisableCoverage=on  SaturateOnIntegerOverflow=on  InputSameDT=on  OutDataTypeStr=Inherit: Same as first input
  Product2 : Product  DisableCoverage=on  SaturateOnIntegerOverflow=on  InputSameDT=on  OutDataTypeStr=Inherit: Same as first input
  Product3 : Product
  Product4 : Product
  Selector : Selector  InputPortWidth=1  IndexOptions=Index vector (dialog)  Indices=[1]  OutputSizes=1
  Sum : Sum  DisableCoverage=on  Inputs=|++  SaturateOnIntegerOverflow=on  InputSameDT=on  OutDataTypeStr=Inherit: Same as first input
  targetTime : Constant  DisableCoverage=on  Value=T
  vib : Outport
  wires:
  Sum/1 -> Product2/2
  targetTime/1 -> Product/2
  Output/1 -> vib/1
  Clock1/1 -> Product2/1, Product1/1
  Gain/1 -> Product1/2
  Product2/1 -> Output/1
  Product/1 -> Gain/1
  Product3/1 -> Product/1
  Product1/1 -> Sum/1
  rpm/1 -> Selector/1, Product3/2
  Constant/1 -> Product3/1
  Selector/1 -> Product4/1
  Constant1/1 -> Product4/2
  Product4/1 -> Sum/2

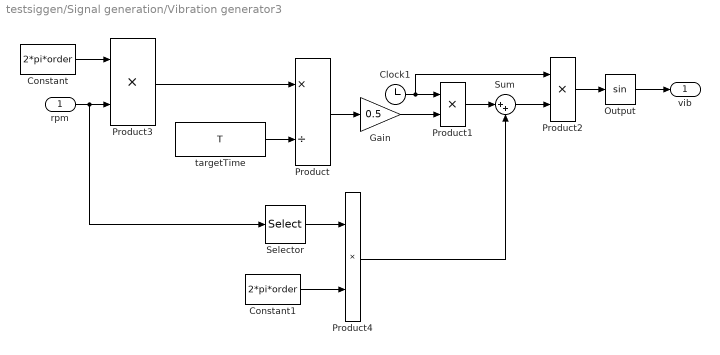
== system testsiggen/Signal generation/Vibration generator3 ==
  rpm : Inport
  Clock1 : Clock
      settings: DisableCoverage=on
  Constant : Constant  Value=2*pi*order
  Constant1 : Constant  Value=2*pi*order
  Gain : Gain  DisableCoverage=on  Gain=0.5  OutDataTypeStr=Inherit: Same as input  ParamDataTypeStr=Inherit: Same as input
  Output : Trigonometry
  Product : Product  DisableCoverage=on  Inputs=*/  SaturateOnIntegerOverflow=on  InputSameDT=on  OutDataTypeStr=Inherit: Same as first input
  Product1 : Product  DisableCoverage=on  SaturateOnIntegerOverflow=on  InputSameDT=on  OutDataTypeStr=Inherit: Same as first input
  Product2 : Product  DisableCoverage=on  SaturateOnIntegerOverflow=on  InputSameDT=on  OutDataTypeStr=Inherit: Same as first input
  Product3 : Product
  Product4 : Product
  Selector : Selector  InputPortWidth=1  IndexOptions=Index vector (dialog)  Indices=[1]  OutputSizes=1
  Sum : Sum  DisableCoverage=on  Inputs=|++  SaturateOnIntegerOverflow=on  InputSameDT=on  OutDataTypeStr=Inherit: Same as first input
  targetTime : Constant  DisableCoverage=on  Value=T
  vib : Outport
  wires:
  Sum/1 -> Product2/2
  targetTime/1 -> Product/2
  Output/1 -> vib/1
  Clock1/1 -> Product2/1, Product1/1
  Gain/1 -> Product1/2
  Product2/1 -> Output/1
  Product/1 -> Gain/1
  Product3/1 -> Product/1
  Product1/1 -> Sum/1
  rpm/1 -> Selector/1, Product3/2
  Constant/1 -> Product3/1
  Selector/1 -> Product4/1
  Constant1/1 -> Product4/2
  Product4/1 -> Sum/2

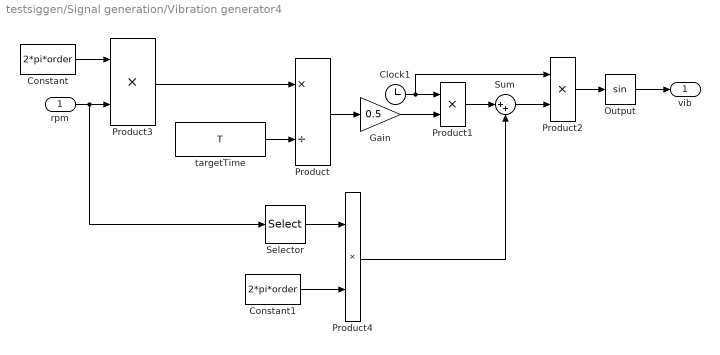
== system testsiggen/Signal generation/Vibration generator4 ==
  rpm : Inport
  Clock1 : Clock
      settings: DisableCoverage=on
  Constant : Constant  Value=2*pi*order
  Constant1 : Constant  Value=2*pi*order
  Gain : Gain  DisableCoverage=on  Gain=0.5  OutDataTypeStr=Inherit: Same as input  ParamDataTypeStr=Inherit: Same as input
  Output : Trigonometry
  Product : Product  DisableCoverage=on  Inputs=*/  SaturateOnIntegerOverflow=on  InputSameDT=on  OutDataTypeStr=Inherit: Same as first input
  Product1 : Product  DisableCoverage=on  SaturateOnIntegerOverflow=on  InputSameDT=on  OutDataTypeStr=Inherit: Same as first input
  Product2 : Product  DisableCoverage=on  SaturateOnIntegerOverflow=on  InputSameDT=on  OutDataTypeStr=Inherit: Same as first input
  Product3 : Product
  Product4 : Product
  Selector : Selector  InputPortWidth=1  IndexOptions=Index vector (dialog)  Indices=[1]  OutputSizes=1
  Sum : Sum  DisableCoverage=on  Inputs=|++  SaturateOnIntegerOverflow=on  InputSameDT=on  OutDataTypeStr=Inherit: Same as first input
  targetTime : Constant  DisableCoverage=on  Value=T
  vib : Outport
  wires:
  Sum/1 -> Product2/2
  targetTime/1 -> Product/2
  Output/1 -> vib/1
  Clock1/1 -> Product2/1, Product1/1
  Gain/1 -> Product1/2
  Product2/1 -> Output/1
  Product/1 -> Gain/1
  Product3/1 -> Product/1
  Product1/1 -> Sum/1
  rpm/1 -> Selector/1, Product3/2
  Constant/1 -> Product3/1
  Selector/1 -> Product4/1
  Constant1/1 -> Product4/2
  Product4/1 -> Sum/2

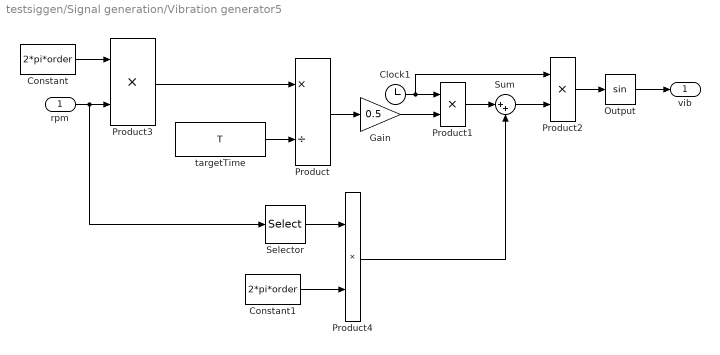
== system testsiggen/Signal generation/Vibration generator5 ==
  rpm : Inport
  Clock1 : Clock
      settings: DisableCoverage=on
  Constant : Constant  Value=2*pi*order
  Constant1 : Constant  Value=2*pi*order
  Gain : Gain  DisableCoverage=on  Gain=0.5  OutDataTypeStr=Inherit: Same as input  ParamDataTypeStr=Inherit: Same as input
  Output : Trigonometry
  Product : Product  DisableCoverage=on  Inputs=*/  SaturateOnIntegerOverflow=on  InputSameDT=on  OutDataTypeStr=Inherit: Same as first input
  Product1 : Product  DisableCoverage=on  SaturateOnIntegerOverflow=on  InputSameDT=on  OutDataTypeStr=Inherit: Same as first input
  Product2 : Product  DisableCoverage=on  SaturateOnIntegerOverflow=on  InputSameDT=on  OutDataTypeStr=Inherit: Same as first input
  Product3 : Product
  Product4 : Product
  Selector : Selector  InputPortWidth=1  IndexOptions=Index vector (dialog)  Indices=[1]  OutputSizes=1
  Sum : Sum  DisableCoverage=on  Inputs=|++  SaturateOnIntegerOverflow=on  InputSameDT=on  OutDataTypeStr=Inherit: Same as first input
  targetTime : Constant  DisableCoverage=on  Value=T
  vib : Outport
  wires:
  Sum/1 -> Product2/2
  targetTime/1 -> Product/2
  Output/1 -> vib/1
  Clock1/1 -> Product2/1, Product1/1
  Gain/1 -> Product1/2
  Product2/1 -> Output/1
  Product/1 -> Gain/1
  Product3/1 -> Product/1
  Product1/1 -> Sum/1
  rpm/1 -> Selector/1, Product3/2
  Constant/1 -> Product3/1
  Selector/1 -> Product4/1
  Constant1/1 -> Product4/2
  Product4/1 -> Sum/2

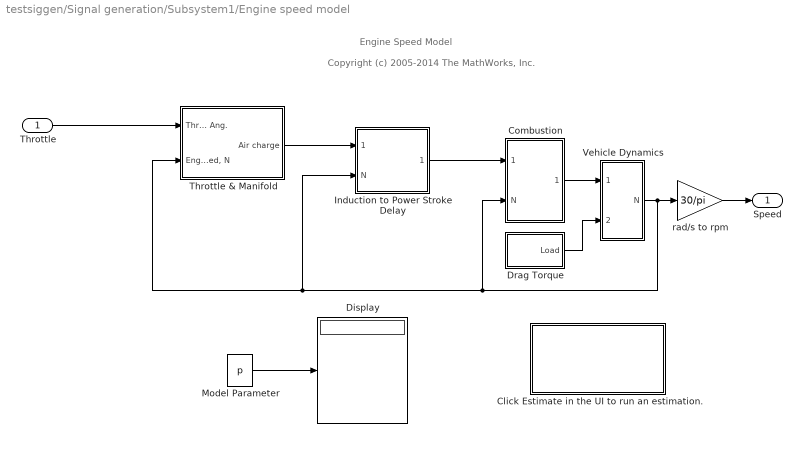
== system testsiggen/Signal generation/Subsystem1/Engine speed model ==
  note: Engine Speed Model
  note: Copyright (c) 2005-2014 The MathWorks, Inc.
  Throttle : Inport
  Click Estimate in the UI to run an estimation. : Subsystem
      settings: OpenFcn=sdotool( slResolve('spe_speed_sdosession', 'spe_speed') );
      mask Display: disp('Parameter Estimation\nwith preloaded data')
  Combustion : Subsystem
  Display : Display
  Drag Torque : Subsystem
  Induction to Power Stroke Delay : Subsystem
  Model Parameter : Constant  Value=p
  Throttle & Manifold : Subsystem
  Vehicle Dynamics : Subsystem
  rad/s to rpm : Gain  Gain=30/pi  SaturateOnIntegerOverflow=on  OutDataTypeStr=Inherit: Same as input  ParamDataTypeStr=Inherit: Same as input
  Speed : Outport
  wires:
  Vehicle Dynamics/1(N) -> rad/s to rpm/1, Combustion/2(N), Throttle & Manifold/2("Engine Speed, N"), Induction to Power Stroke Delay/2(N)
  Drag Torque/1(Load) -> Vehicle Dynamics/2(Tload)
  Combustion/1(Torque) -> Vehicle Dynamics/1(Teng)
  Model Parameter/1 -> Display/1
  Induction to Power Stroke Delay/1(Air Charge) -> Combustion/1(Air Charge)
  Throttle & Manifold/1(Air charge) -> Induction to Power Stroke Delay/1(Air charge)
  Throttle/1 -> Throttle & Manifold/1(Throttle Ang.)
  rad/s to rpm/1 -> Speed/1

== system testsiggen/Signal generation/Subsystem1/Engine speed model/Click Estimate in the UI to run an estimation. ==

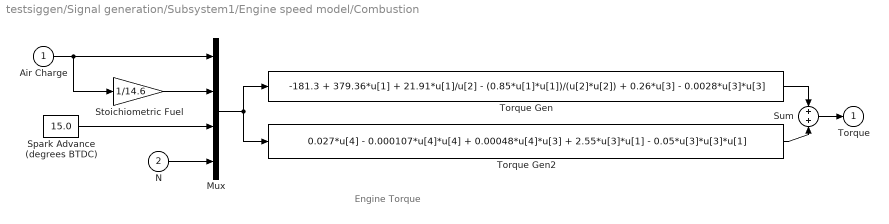
== system testsiggen/Signal generation/Subsystem1/Engine speed model/Combustion ==
  note: Engine Torque
  Air Charge : Inport
  N : Inport  Port=2
  Mux : Mux
  Spark Advance (degrees BTDC) : Constant  Value=15.0
  Stoichiometric Fuel : Gain  Gain=1/14.6  SaturateOnIntegerOverflow=on  OutDataTypeStr=Inherit: Same as input  ParamDataTypeStr=Inherit: Same as input
  Sum : Sum  SaturateOnIntegerOverflow=on  InputSameDT=on  OutDataTypeStr=Inherit: Same as first input
  Torque Gen : Fcn  Expr=-181.3 + 379.36*u[1] + 21.91*u[1]/u[2] - (0.85*u[1]*u[1])/(u[2]*u[2]) + 0.26*u[3] - 0.0028*u[3]*u[3]
  Torque Gen2 : Fcn  Expr=0.027*u[4] - 0.000107*u[4]*u[4] + 0.00048*u[4]*u[3] + 2.55*u[3]*u[1] - 0.05*u[3]*u[3]*u[1]
  Torque : Outport  InitialOutput=0
  wires:
  Stoichiometric Fuel/1 -> Mux/2
  Spark Advance (degrees BTDC)/1 -> Mux/3
  N/1 -> Mux/4
  Air Charge/1 -> Stoichiometric Fuel/1, Mux/1
  Mux/1 -> Torque Gen/1, Torque Gen2/1
  Torque Gen2/1 -> Sum/2
  Torque Gen/1 -> Sum/1
  Sum/1 -> Torque/1

== system testsiggen/Signal generation/Subsystem1/Engine speed model/Drag Torque ==
  note: Torque Disturbances
  Step : Step  Time=2  Before=25  After=25  SampleTime=0
  Step1 : Step  Time=8  After=0  SampleTime=0
  Sum1 : Sum  SaturateOnIntegerOverflow=on  InputSameDT=on  OutDataTypeStr=Inherit: Same as first input
  Load : Outport  InitialOutput=0
  wires:
  Step1/1 -> Sum1/2
  Step/1 -> Sum1/1
  Sum1/1 -> Load/1

== system testsiggen/Signal generation/Subsystem1/Engine speed model/Induction to Power Stroke Delay ==
  Air charge : Inport
  N : Inport  Port=2
  Constant : Constant  Value=pi
  Divide : Product  Inputs=/*
  dM/dt delay : VariableTransportDelay  MaximumDelay=20  InitialOutput=0.152  MaximumPoints=3072  ZeroDelay=on  PadeOrder=2
  Air Charge : Outport
  wires:
  dM/dt delay/1 -> Air Charge/1
  Constant/1 -> Divide/2
  Divide/1 -> dM/dt delay/2
  Air charge/1 -> dM/dt delay/1
  N/1 -> Divide/1

== system testsiggen/Signal generation/Subsystem1/Engine speed model/Throttle & Manifold ==
  note: Air Intake Dynamics
  Throttle Ang. : Inport
  "Engine Speed, N" : Inport  Port=2
  0 <= theta <= 90 : Saturate  UpperLimit=90  LowerLimit=0
  "Atmospheric Pressure, Pa (bar)" : Constant  Value=1.0
  Intake Manifold : Subsystem
  Throttle : Subsystem
  Air charge : Outport  InitialOutput=0
  wires:
  "Atmospheric Pressure, Pa (bar)"/1 -> Throttle/3("Atmospheric Pressure, Pa (bar) ")
  Intake Manifold/1(Air charge) -> Air charge/1
  Intake Manifold/2("Manifold Pressure, Pm (bar)") -> Throttle/2("Manifold Pressure, Pm (bar)")
  "Engine Speed, N"/1 -> Intake Manifold/2(N (rad/sec))
  Throttle/1("Throttle Flow, mdot (g/s)") -> Intake Manifold/1(mdot Input (g/s))
  Throttle Ang./1 -> 0 <= theta <= 90/1
  0 <= theta <= 90/1 -> Throttle/1("Throttle Angle, theta (deg)")

== system testsiggen/Signal generation/Subsystem1/Engine speed model/Vehicle Dynamics ==
  Teng : Inport
  Tload : Inport  Port=2
  Constant1 : Constant  Value=10
  "Inverse Inertia, 1/J" : Gain  Gain=1/J  SaturateOnIntegerOverflow=on  OutDataTypeStr=Inherit: Same as input  ParamDataTypeStr=Inherit: Same as input
  MinMax : MinMax  Function=max  Inputs=2
  Sum : Sum  Inputs=+-  SaturateOnIntegerOverflow=on  InputSameDT=on  OutDataTypeStr=Inherit: Same as first input
  engine speed : Integrator  InitialCondition=209.48
  N : Outport  InitialOutput=0
  wires:
  "Inverse Inertia, 1/J"/1 -> engine speed/1
  Sum/1 -> "Inverse Inertia, 1/J"/1
  Teng/1 -> Sum/1
  Tload/1 -> Sum/2
  MinMax/1 -> N/1
  engine speed/1 -> MinMax/1
  Constant1/1 -> MinMax/2

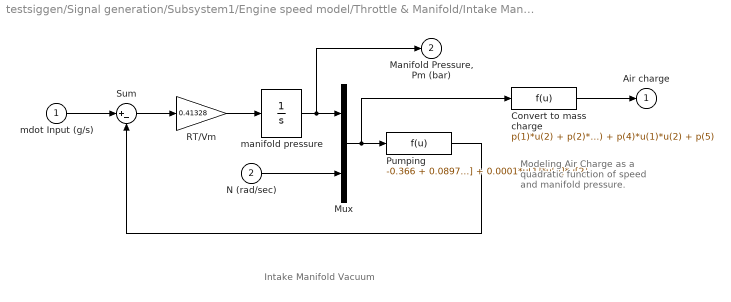
== system testsiggen/Signal generation/Subsystem1/Engine speed model/Throttle & Manifold/Intake Manifold ==
  note: Intake Manifold Vacuum
  note: Modeling Air Charge as a
      | quadratic function of speed
      | and manifold pressure.
  mdot Input (g/s) : Inport
  N (rad/sec) : Inport  Port=2
  Convert to mass charge : Fcn  Expr=p(1)*u(2) + p(2)*u(1) + p(3)*u(1)*u(1) + p(4)*u(1)*u(2) + p(5)
  Mux : Mux  Inputs=2
  Pumping : Fcn  Expr=-0.366 + 0.08979*u[1]*u[2] - 0.0337*u[2]*u[1]*u[1] + 0.0001*u[1]*u[2]*u[2]
  RT/Vm : Gain  Gain=0.41328  SaturateOnIntegerOverflow=on  OutDataTypeStr=Inherit: Same as input  ParamDataTypeStr=Inherit: Same as input
  Sum : Sum  Inputs=|+-  SaturateOnIntegerOverflow=on  InputSameDT=on  OutDataTypeStr=Inherit: Same as first input
  manifold pressure : Integrator  InitialCondition=0.543
  Air charge : Outport  InitialOutput=0
  "Manifold Pressure, Pm (bar)" : Outport  Port=2  InitialOutput=0
  wires:
  Pumping/1 -> Sum/2
  Sum/1 -> RT/Vm/1
  manifold pressure/1 -> "Manifold Pressure, Pm (bar)"/1, Mux/1
  Mux/1 -> Pumping/1, Convert to mass charge/1
  N (rad/sec)/1 -> Mux/2
  RT/Vm/1 -> manifold pressure/1
  mdot Input (g/s)/1 -> Sum/1
  Convert to mass charge/1 -> Air charge/1

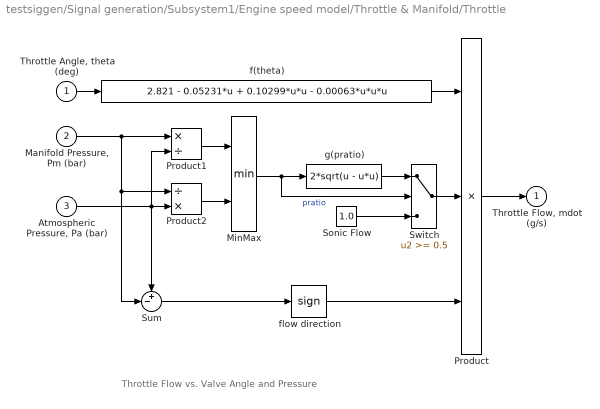
== system testsiggen/Signal generation/Subsystem1/Engine speed model/Throttle & Manifold/Throttle ==
  note: Throttle Flow vs. Valve Angle and Pressure
  "Throttle Angle, theta (deg)" : Inport
  "Manifold Pressure, Pm (bar)" : Inport  Port=2
  "Atmospheric Pressure, Pa (bar) " : Inport  Port=3
  MinMax : MinMax  Inputs=2  SaturateOnIntegerOverflow=on  InputSameDT=on
  Product : Product  Inputs=3  SaturateOnIntegerOverflow=on  RndMeth=Zero  InputSameDT=on  OutDataTypeStr=Inherit: Same as first input
  Product1 : Product  Inputs=*/  SaturateOnIntegerOverflow=on  RndMeth=Zero  InputSameDT=on  OutDataTypeStr=Inherit: Same as first input
  Product2 : Product  Inputs=/*  SaturateOnIntegerOverflow=on  RndMeth=Zero  InputSameDT=on  OutDataTypeStr=Inherit: Same as first input
  "Sonic Flow " : Constant  Value=1.0
  Sum : Sum  Inputs=+-|  SaturateOnIntegerOverflow=on  InputSameDT=on  OutDataTypeStr=Inherit: Same as first input
  Switch : Switch  Threshold=0.5  SaturateOnIntegerOverflow=on  InputSameDT=on
  f(theta) : Fcn  Expr=2.821 - 0.05231*u + 0.10299*u*u - 0.00063*u*u*u
  flow direction : Signum
  g(pratio) : Fcn  Expr=2*sqrt(u - u*u)
  "Throttle Flow, mdot (g/s)" : Outport  InitialOutput=0
  wires:
  f(theta)/1 -> Product/1
  Product/1 -> "Throttle Flow, mdot (g/s)"/1
  "Throttle Angle, theta (deg)"/1 -> f(theta)/1
  MinMax/1 -> g(pratio)/1, Switch/2  "pratio"
  Sum/1 -> flow direction/1
  flow direction/1 -> Product/3
  Switch/1 -> Product/2
  "Sonic Flow "/1 -> Switch/3
  g(pratio)/1 -> Switch/1
  "Atmospheric Pressure, Pa (bar) "/1 -> Product1/2, Product2/2, Sum/1
  Product1/1 -> MinMax/1
  Product2/1 -> MinMax/2
  "Manifold Pressure, Pm (bar)"/1 -> Product1/1, Product2/1, Sum/2
